simulink model "s_qube2_bal_rl"  (R2021a)
settings: Solver=ode1  StartTime=0.0  StopTime=Tf  FixedStep=Ts  MaxStep=0.02  MinStep=0.001  RelTol=1e-3  EnableMultiTasking=on
undefined symbols (not defined in the file or in its folder): alpha_bal_threshold, B, bp, br, g, ic_alpha0, Jp, Jr, km, kt, l, mp, q11, q22, q33, q44, r, Rm, theta_max, Vmax
libraries: simulink x3, simulink_extras x2, rllib x1
settings Model: ExtModeTrigDuration=5000  OrderedModelArguments=off  Creator=MLevis  LastModifiedBy=MLevis
settings SolverCC: InitialStep=Ts  AlgebraicLoopSolver=TrustRegion
settings DebuggingCC: UnderspecifiedInitializationDetection=Classic  MergeDetectMultiDrivingBlocksExec=none  SFMachineParentedDataDiag=warning
settings ModelReferenceCC: PropagateSignalLabelsOutOfModel=off
settings SFSimCC: CustomCodeUndefinedFunction=UseInterfaceOnly

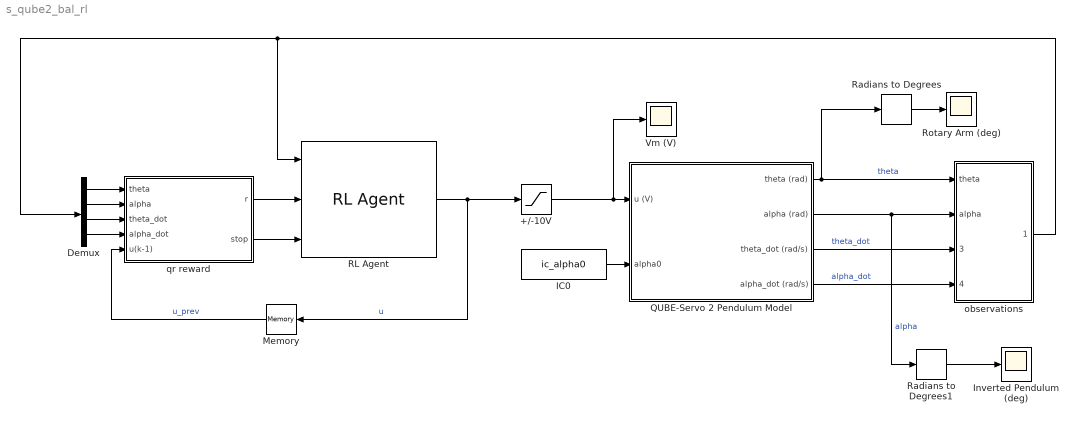
== system s_qube2_bal_rl ==
  +/-10V : Saturate  UpperLimit=Vmax  LowerLimit=-Vmax  OutDataTypeStr=Inherit: Inherit via back propagation
  Demux : Demux
  IC0 : Constant  Value=ic_alpha0
  Inverted Pendulum (deg) : Scope
  Memory : Memory
  QUBE-Servo 2 Pendulum Model : Subsystem
  RL Agent : rllib/RL Agent  Agent=agent  ExternalActionAsInput=off  ProvideCumRwd=off  TreatAsDirectFeedthrough=on
  Radians to Degrees : simulink_extras/Transformations/Radians to Degrees
  Radians to Degrees1 : simulink_extras/Transformations/Radians to Degrees
  Rotary Arm (deg) : Scope
  Vm (V) : Scope
  observations : Subsystem  VariantControl=sincos
  qr reward : Subsystem
  wires:
  Radians to Degrees/1 -> Rotary Arm (deg)/1
  Radians to Degrees1/1 -> Inverted Pendulum (deg)/1
  +/-10V/1 -> QUBE-Servo 2 Pendulum Model/1(u (V)), Vm (V)/1
  RL Agent/1 -> +/-10V/1, Memory/1  "u"
  QUBE-Servo 2 Pendulum Model/2(alpha (rad)) -> Radians to Degrees1/1, observations/2(alpha)  "alpha"
  QUBE-Servo 2 Pendulum Model/1(theta (rad)) -> Radians to Degrees/1, observations/1(theta)  "theta"
  QUBE-Servo 2 Pendulum Model/3(theta_dot (rad/s)) -> observations/3(theta_dot)  "theta_dot"
  QUBE-Servo 2 Pendulum Model/4(alpha_dot (rad/s)) -> observations/4(alpha_dot)  "alpha_dot"
  qr reward/1(r) -> RL Agent/2
  IC0/1 -> QUBE-Servo 2 Pendulum Model/2(alpha0)
  qr reward/2(stop) -> RL Agent/3
  Demux/1 -> qr reward/1(theta)
  Demux/2 -> qr reward/2(alpha)
  Demux/3 -> qr reward/3(theta_dot)
  Demux/4 -> qr reward/4(alpha_dot)
  Memory/1 -> qr reward/5(u(k-1))  "u_prev"
  observations/1(observations) -> RL Agent/1, Demux/1

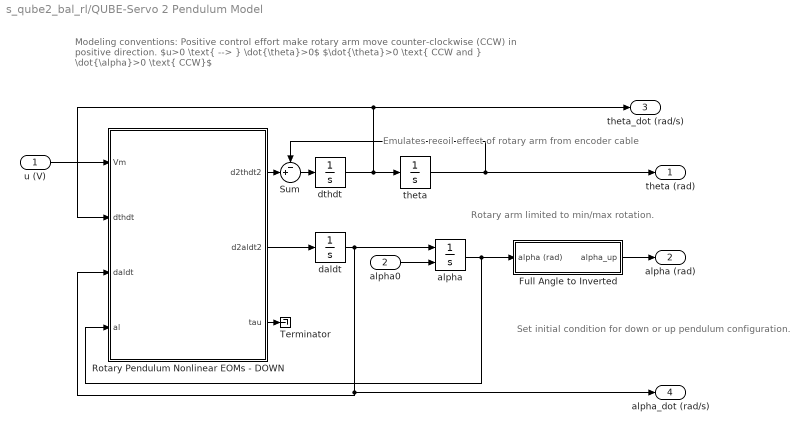
== system s_qube2_bal_rl/QUBE-Servo 2 Pendulum Model ==
  note: Rotary arm limited to min/max rotation.
  note: Modeling conventions:
      | Positive control effort make rotary arm move counter-clockwise (CCW) in positive direction.
      | $u>0 \text{ --> } \dot{\theta}>0$
      | $\dot{\theta}>0 \text{ CCW and } \dot{\alpha}>0 \text{ CCW}$
  note: Set initial condition for down or up pendulum configuration.
  note: Emulates recoil effect of rotary arm from encoder cable
  u (V) : Inport
  alpha0 : Inport  Port=2
  Full Angle to Inverted : Subsystem
  Rotary Pendulum Nonlinear EOMs - DOWN : MATLAB Function  TreatAsAtomicUnit=on
  Sum : Sum  Inputs=-+|
  Terminator : Terminator
  alpha : Integrator  InitialConditionSource=external  InitialCondition=ic_alpha0
  daldt : Integrator
  dthdt : Integrator
  theta : Integrator  LimitOutput=on  UpperSaturationLimit=theta_max  LowerSaturationLimit=-theta_max
  theta (rad) : Outport  VectorParamsAs1DForOutWhenUnconnected=off
  alpha (rad) : Outport  Port=2  VectorParamsAs1DForOutWhenUnconnected=off
  theta_dot (rad/s) : Outport  Port=3  VectorParamsAs1DForOutWhenUnconnected=off
  alpha_dot (rad/s) : Outport  Port=4  VectorParamsAs1DForOutWhenUnconnected=off
  wires:
  daldt/1 -> Rotary Pendulum Nonlinear EOMs - DOWN/3(daldt), alpha_dot (rad/s)/1, alpha/1
  alpha/1 -> Full Angle to Inverted/1(alpha (rad)), Rotary Pendulum Nonlinear EOMs - DOWN/4(al)
  Rotary Pendulum Nonlinear EOMs - DOWN/2(d2aldt2) -> daldt/1
  dthdt/1 -> theta_dot (rad/s)/1, Rotary Pendulum Nonlinear EOMs - DOWN/2(dthdt), theta/1
  u (V)/1 -> Rotary Pendulum Nonlinear EOMs - DOWN/1(Vm)
  Rotary Pendulum Nonlinear EOMs - DOWN/3(tau) -> Terminator/1
  Full Angle to Inverted/1(alpha_up) -> alpha (rad)/1
  alpha0/1 -> alpha/2
  theta/1 -> theta (rad)/1, Sum/1
  Rotary Pendulum Nonlinear EOMs - DOWN/1(d2thdt2) -> Sum/2
  Sum/1 -> dthdt/1

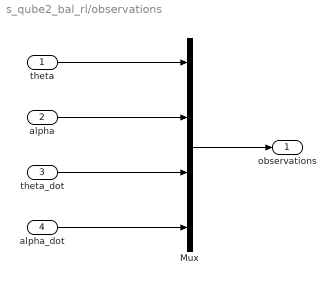
== system s_qube2_bal_rl/observations ==
  theta : Inport
  alpha : Inport  Port=2
  theta_dot : Inport  Port=3
  alpha_dot : Inport  Port=4
  Mux : Mux
  observations : Outport  VectorParamsAs1DForOutWhenUnconnected=off
  wires:
  theta/1 -> Mux/1
  alpha/1 -> Mux/2
  Mux/1 -> observations/1
  theta_dot/1 -> Mux/3
  alpha_dot/1 -> Mux/4

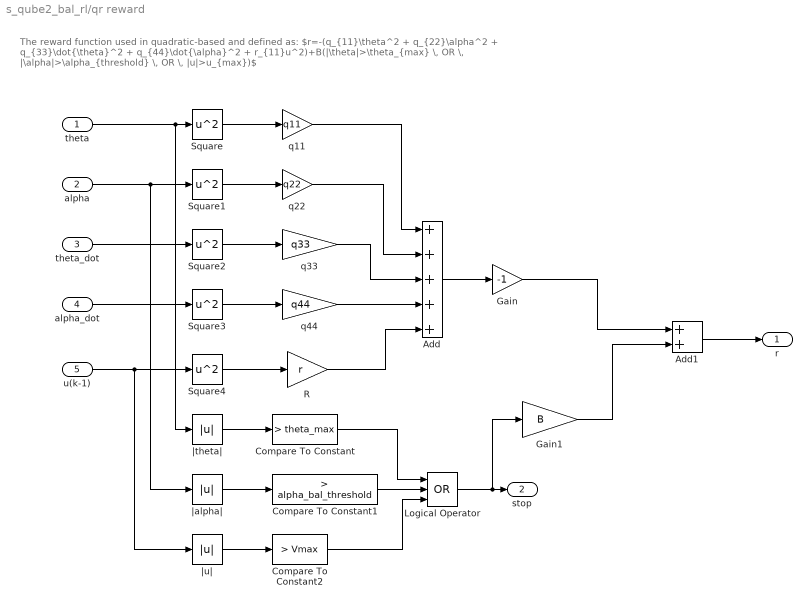
== system s_qube2_bal_rl/qr reward ==
  note: The reward function used in quadratic-based and defined as:
      | $r=-(q_{11}\theta^2 + q_{22}\alpha^2 + q_{33}\dot{\theta}^2 + q_{44}\dot{\alpha}^2 + r_{11}u^2)+B(|\theta|>\theta_{max} \, OR \, |\alpha|>\alpha_{threshold} \, OR \, |u|>u_{max})$
  theta : Inport
  alpha : Inport  Port=2
  theta_dot : Inport  Port=3
  alpha_dot : Inport  Port=4
  u(k-1) : Inport  Port=5
  Add : Sum  Inputs=+++++
  Add1 : Sum
  Compare To Constant : simulink/Logic and Bit Operations/Compare To Constant  relop=>  const=theta_max  OutDataTypeStr=boolean
  Compare To Constant1 : simulink/Logic and Bit Operations/Compare To Constant  relop=>  const=alpha_bal_threshold  OutDataTypeStr=boolean
  Compare To Constant2 : simulink/Logic and Bit Operations/Compare To Constant  relop=>  const=Vmax  OutDataTypeStr=boolean
  Gain : Gain  Gain=-1
  Gain1 : Gain  Gain=B
  Logical Operator : Logic  Operator=OR  Inputs=3  AllPortsSameDT=off  OutDataTypeStr=boolean
  R : Gain  Gain=r
  Square{,1..4} (5 alike) : Math  Operator=square  SaturateOnIntegerOverflow=on
  q11 : Gain  Gain=q11
  q22 : Gain  Gain=q22
  q33 : Gain  Gain=q33
  q44 : Gain  Gain=q44
  |alpha| : Abs
  |theta| : Abs
  |u| : Abs
  r : Outport  VectorParamsAs1DForOutWhenUnconnected=off
  stop : Outport  Port=2  VectorParamsAs1DForOutWhenUnconnected=off
  wires:
  |theta|/1 -> Compare To Constant/1
  theta/1 -> Square/1, |theta|/1
  Compare To Constant/1 -> Logical Operator/1
  alpha/1 -> Square1/1, |alpha|/1
  |alpha|/1 -> Compare To Constant1/1
  Logical Operator/1 -> Gain1/1, stop/1
  Square/1 -> q11/1
  Square1/1 -> q22/1
  Square2/1 -> q33/1
  theta_dot/1 -> Square2/1
  alpha_dot/1 -> Square3/1
  Square3/1 -> q44/1
  u(k-1)/1 -> Square4/1, |u|/1
  Square4/1 -> R/1
  |u|/1 -> Compare To Constant2/1
  R/1 -> Add/5
  q11/1 -> Add/1
  q33/1 -> Add/3
  q22/1 -> Add/2
  q44/1 -> Add/4
  Add/1 -> Gain/1
  Compare To Constant2/1 -> Logical Operator/3
  Compare To Constant1/1 -> Logical Operator/2
  Gain/1 -> Add1/1
  Gain1/1 -> Add1/2
  Add1/1 -> r/1

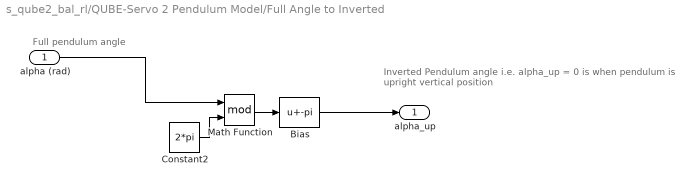
== system s_qube2_bal_rl/QUBE-Servo 2 Pendulum Model/Full Angle to Inverted ==
  note: Inverted Pendulum angle
      | i.e. alpha_up = 0 is when pendulum is upright vertical position
  note: Full pendulum angle
  alpha (rad) : Inport
  Bias : Bias  Bias=-pi
  Constant2 : Constant  Value=2*pi
  Math Function : Math  Operator=mod  SignedPower=on  SaturateOnIntegerOverflow=on
  alpha_up : Outport  VectorParamsAs1DForOutWhenUnconnected=off
  wires:
  Constant2/1 -> Math Function/2
  Bias/1 -> alpha_up/1
  alpha (rad)/1 -> Math Function/1
  Math Function/1 -> Bias/1

== matlab function s_qube2_bal_rl/QUBE-Servo 2 Pendulum Model/Rotary Pendulum Nonlinear EOMs - DOWN ==
  data: Vm input size=1; d2thdt2 output size=1; d2aldt2 output size=1; dthdt input size=1; daldt input size=1; Jp parameter; Jr parameter; l parameter; mp parameter; br parameter; bp parameter; r parameter; kt parameter; km parameter; Rm parameter; al input size=1; g parameter; tau output
function [d2thdt2,d2aldt2,tau] = pen_nonlin_eoms(Vm, dthdt, daldt, Jp, Jr, l, mp, br, bp, r, kt, km, Rm, al, g)

% Convert voltage to torque input
tau = (Vm - km*dthdt)/Rm;
tau=kt*tau;
% Denominator
Jt = Jr*Jp + Jp^2*sin(al)^2 - mp^2*r^2*l^2*cos(al)^2;
% Nonlinear equations of motion for generic rotary pendulum (i.e. furuta)
% Terms from EOM solving
term1 = tau - br*dthdt + 2*Jp*sin(al)*cos(al)*dthdt*daldt + mp*r*l*sin(al)*daldt^2;
term2 = -bp*daldt - Jp*sin(al)*cos(al)*daldt^2 - mp*g*l*sin(al);
% Torque to rotary arm position)
d2thdt2 = 1/Jt*( Jp*term1 - mp*r*l*cos(al)*term2);
% Torque to pendulum angle position
d2aldt2 = 1/Jt*(-mp*r*l*cos(al)*term1 + (Jr+Jp*sin(al)^2)*term2);
